simulink model "QPSK_mod_demod"  (R2020b)
settings: Solver=VariableStepAuto  StartTime=0.0  StopTime=0  RelTol=1e-3
libraries: dspsrcs4 x4, simulink x3, dsparch4 x2, commseqgen3 x2
settings Model: Creator=Mohit Akhouri  LastModifiedBy=Mohit Akhouri

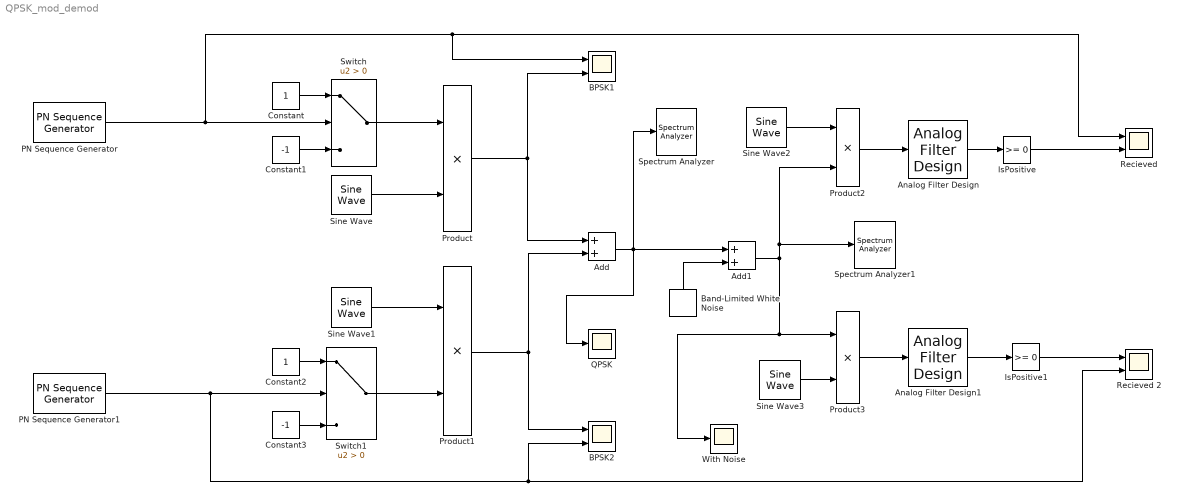
== system QPSK_mod_demod ==
  Add : Sum
  Add1 : Sum
  Analog Filter Design : dsparch4/Analog Filter Design  method=Butterworth  filttype=Lowpass  N=8  Wlo=2*pi*1000  Whi=80  Rp=2  Rs=40
  Analog Filter Design1 : dsparch4/Analog Filter Design  method=Butterworth  filttype=Lowpass  N=8  Wlo=2*pi*1000  Whi=80  Rp=2  Rs=40
  BPSK1 : Scope  NumInputPorts=2
  BPSK2 : Scope  NumInputPorts=2
  Band-Limited White Noise : simulink/Sources/Band-Limited White Noise  Cov=[0.00001]  Ts=0.001  seed=[23341]
  Constant : Constant
  Constant1 : Constant  Value=-1
  Constant2 : Constant
  Constant3 : Constant  Value=-1
  IsPositive : simulink/Logic and Bit Operations/Compare To Zero  relop=>=  OutDataTypeStr=boolean
  IsPositive1 : simulink/Logic and Bit Operations/Compare To Zero  relop=>=  OutDataTypeStr=boolean
  PN Sequence Generator : commseqgen3/PN Sequence Generator  poly='z^6 + z^3 + 1'  ini_sta=[0 0 0 0 0 1]  outBitMaskSource=Dialog parameter  shift=0  outVarSiz=off  maxOutSizeMode=Dialog parameter  maxOutSize=[10 1]  Ts=0.001  sampPerFrame=1  reset=off  bitPackedOutputs=off  outDataType=double  numPackedBits=8  bitPackDataSigned=off  bitPackedOutDType=double
  PN Sequence Generator1 : commseqgen3/PN Sequence Generator  poly='z^6 + z^5 + 1'  ini_sta=[0 0 0 0 0 1]  outBitMaskSource=Dialog parameter  shift=0  outVarSiz=off  maxOutSizeMode=Dialog parameter  maxOutSize=[10 1]  Ts=0.001  sampPerFrame=1  reset=off  bitPackedOutputs=off  outDataType=double  numPackedBits=8  bitPackDataSigned=off  bitPackedOutDType=double
  Product{,1..3} (4 alike) : Product
  QPSK : Scope
  Recieved : Scope  NumInputPorts=2
  "Recieved 2 " : Scope  NumInputPorts=2
  Sine Wave : dspsrcs4/Sine Wave  Amplitude=1  Frequency=1000  Phase=0  SampleMode=Discrete  OutComplex=Real  CompMethod=Trigonometric fcn  TableSize=Speed  SampleTime=1/1000000  SamplesPerFrame=1  ResetState=Restart at time zero  OutputFrames=off  dataType=double  wordLen=16  udDataType=sfix(16)  fracBitsMode=Best precision  numFracBits=15  OutDataTypeStr=double  LastOutDataTypeStr=double
  Sine Wave1 : dspsrcs4/Sine Wave  Amplitude=1  Frequency=1000  Phase=pi/2  SampleMode=Discrete  OutComplex=Real  CompMethod=Trigonometric fcn  TableSize=Speed  SampleTime=1/1000000  SamplesPerFrame=1  ResetState=Restart at time zero  OutputFrames=off  dataType=double  wordLen=16  udDataType=sfix(16)  fracBitsMode=Best precision  numFracBits=15  OutDataTypeStr=double  LastOutDataTypeStr=double
  Sine Wave2 : dspsrcs4/Sine Wave  Amplitude=1  Frequency=1000  Phase=0  SampleMode=Discrete  OutComplex=Real  CompMethod=Trigonometric fcn  TableSize=Speed  SampleTime=1/1000000  SamplesPerFrame=1  ResetState=Restart at time zero  OutputFrames=off  dataType=double  wordLen=16  udDataType=sfix(16)  fracBitsMode=Best precision  numFracBits=15  OutDataTypeStr=double  LastOutDataTypeStr=double
  Sine Wave3 : dspsrcs4/Sine Wave  Amplitude=1  Frequency=1000  Phase=pi/2  SampleMode=Discrete  OutComplex=Real  CompMethod=Trigonometric fcn  TableSize=Speed  SampleTime=1/1000000  SamplesPerFrame=1  ResetState=Restart at time zero  OutputFrames=off  dataType=double  wordLen=16  udDataType=sfix(16)  fracBitsMode=Best precision  numFracBits=15  OutDataTypeStr=double  LastOutDataTypeStr=double
  Spectrum Analyzer : SpectrumAnalyzer
  Spectrum Analyzer1 : SpectrumAnalyzer
  Switch : Switch  Criteria=u2 > Threshold
  Switch1 : Switch  Criteria=u2 > Threshold
  With Noise : Scope
  wires:
  Add1/1 -> Spectrum Analyzer1/1, Product2/2, Product3/1, With Noise/1
  Product3/1 -> Analog Filter Design1/1
  PN Sequence Generator/1 -> Recieved/1, BPSK1/1, Switch/2
  Band-Limited White Noise/1 -> Add1/2
  IsPositive/1 -> Recieved/2
  Constant3/1 -> Switch1/3
  Sine Wave2/1 -> Product2/1
  Product/1 -> Add/1, BPSK1/2
  IsPositive1/1 -> "Recieved 2 "/1
  Product2/1 -> Analog Filter Design/1
  Analog Filter Design1/1 -> IsPositive1/1
  Sine Wave3/1 -> Product3/2
  Constant2/1 -> Switch1/1
  Add/1 -> QPSK/1, Spectrum Analyzer/1, Add1/1
  PN Sequence Generator1/1 -> BPSK2/2, "Recieved 2 "/2, Switch1/2
  Switch1/1 -> Product1/2
  Product1/1 -> BPSK2/1, Add/2
  Switch/1 -> Product/1
  Analog Filter Design/1 -> IsPositive/1
  Sine Wave1/1 -> Product1/1
  Sine Wave/1 -> Product/2
  Constant/1 -> Switch/1
  Constant1/1 -> Switch/3
